simulink model "LQR01"  (Simulink 9.2)
settings: Solver=VariableStepAuto  StartTime=0.0  StopTime=60  RelTol=1e-3
libraries: Solver_SF x1, simulink x1
settings Model: Creator=GTR  LastModifiedBy=tomoyo
settings SolverCC: AlgebraicLoopSolver=LineSearch
settings DataIOCC: LimitDataPoints=off  SaveFormat=Dataset  SignalLoggingSaveFormat=Dataset
settings OptimizationCC: LifeSpan=auto
settings DebuggingCC: UnderspecifiedInitializationDetection=Simplified  MergeDetectMultiDrivingBlocksExec=error  FcnCallInpInsideContextMsg=error  StateNameClashWarn=none  SFUnexpectedBacktrackingDiag=error  SFNoUnconditionalDefaultTransitionDiag=error  SFExecutionAtInitializationDiag=warning
settings HardwareCC: ProdBitPerPointer=64  ProdBitPerSizeT=64  ProdBitPerPtrDiffT=64  ProdLargestAtomicFloat=Float  ProdIntDivRoundTo=Zero  ProdEndianess=LittleEndian  ProdWordSize=64  ProdHWDeviceType=Intel->x86-64 (Windows64)
settings ModelReferenceCC: PropagateSignalLabelsOutOfModel=on
settings SFSimCC: SimUseLocalCustomCode=on
settings RTWCC: RTWUseLocalCustomCode=on
settings CodeAppCC: StateflowObjectComments=off
settings GRTTargetCC: TargetLangStandard=C99 (ISO)  GeneratePreprocessorConditionals=Use local settings  CombineOutputUpdateFcns=on  GRTInterface=off
settings ConfigComp: CovMetricSettings=dwe  CovHtmlReporting=off  CovSaveCumulativeToWorkspaceVar=off  CovSaveSingleToWorkspaceVar=off  CovExternalEMLEnable=on

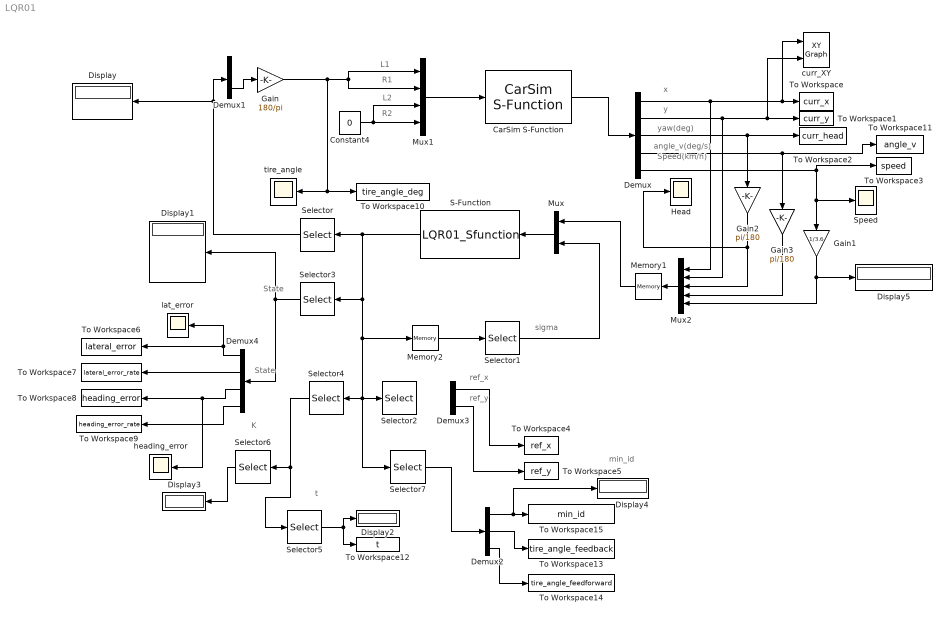
== system LQR01 ==
  note: min_id
  note: K
  note: State
  note: ref_x
  note: sigma
  note: x
  note: y
  note: yaw(deg)
  note: Speed(km/h)
  note: L1
  note: R1
  note: L2
  note: R2
  note: ref_y
  note: State
  note: angle_v(deg/s)
  note: t
  CarSim S-Function : Solver_SF/CarSim S-Function  Priority=1  VehicleCode=i_i  SIMFILE=simfile
  Constant4 : Constant  Value=0
  Demux : Demux  Outputs=5
  Demux1 : Demux  Outputs=2
  Demux2 : Demux  Outputs=3
  Demux3 : Demux  Outputs=2
  Demux4 : Demux
  Display{,1..5} (6 alike) : Display
  Gain : Gain  Gain=180/pi
  Gain1 : Gain  Gain=1/3.6
  Gain2 : Gain  Gain=pi/180
  Gain3 : Gain  Gain=pi/180
  Head : Scope
  Memory1 : Memory
  Memory2 : Memory
  Mux : Mux  Inputs=2
  Mux1 : Mux
  Mux2 : Mux  Inputs=5
  S-Function : S-Function  FunctionName=LQR01_Sfunction  SFunctionDeploymentMode=off  EnableBusSupport=off
  Selector : Selector  InputPortWidth=19  IndexOptions=Index vector (dialog)  Indices=[1 2]  OutputSizes=1
  Selector1 : Selector  InputPortWidth=19  IndexOptions=Index vector (dialog)  Indices=[2]  OutputSizes=1
  Selector2 : Selector  InputPortWidth=19  IndexOptions=Index vector (dialog)  Indices=[6 7]  OutputSizes=1
  Selector3 : Selector  InputPortWidth=19  IndexOptions=Index vector (dialog)  Indices=[8 9 10 11]  OutputSizes=1
  Selector4 : Selector  InputPortWidth=19  IndexOptions=Index vector (dialog)  Indices=[12 13 14 15 16]  OutputSizes=1
  Selector5 : Selector  InputPortWidth=5  IndexOptions=Index vector (dialog)  Indices=[5]  OutputSizes=1
  Selector6 : Selector  InputPortWidth=5  IndexOptions=Index vector (dialog)  Indices=[1 2 3 4]  OutputSizes=1
  Selector7 : Selector  InputPortWidth=19  IndexOptions=Index vector (dialog)  Indices=[17 18 19]  OutputSizes=1
  Speed : Scope
  To Workspace : ToWorkspace  VariableName=curr_x  SaveFormat=Timeseries  SampleTime=-1
  To Workspace1 : ToWorkspace  VariableName=curr_y  SaveFormat=Timeseries  SampleTime=-1
  To Workspace10 : ToWorkspace  VariableName=tire_angle_deg  SaveFormat=Timeseries  SampleTime=-1
  To Workspace11 : ToWorkspace  VariableName=angle_v  SaveFormat=Timeseries  SampleTime=-1
  To Workspace12 : ToWorkspace  VariableName=t  SaveFormat=Timeseries  SampleTime=-1
  To Workspace13 : ToWorkspace  VariableName=tire_angle_feedback  SaveFormat=Timeseries  SampleTime=-1
  To Workspace14 : ToWorkspace  VariableName=tire_angle_feedforward  SaveFormat=Timeseries  SampleTime=-1
  To Workspace15 : ToWorkspace  VariableName=min_id  SaveFormat=Timeseries  SampleTime=-1
  To Workspace2 : ToWorkspace  VariableName=curr_head  SaveFormat=Timeseries  SampleTime=-1
  To Workspace3 : ToWorkspace  VariableName=speed  SaveFormat=Timeseries  SampleTime=-1
  To Workspace4 : ToWorkspace  VariableName=ref_x  SaveFormat=Timeseries  SampleTime=-1
  To Workspace5 : ToWorkspace  VariableName=ref_y  SaveFormat=Timeseries  SampleTime=-1
  To Workspace6 : ToWorkspace  VariableName=lateral_error  SaveFormat=Timeseries  SampleTime=-1
  To Workspace7 : ToWorkspace  VariableName=lateral_error_rate  SaveFormat=Timeseries  SampleTime=-1
  To Workspace8 : ToWorkspace  VariableName=heading_error  SaveFormat=Timeseries  SampleTime=-1
  To Workspace9 : ToWorkspace  VariableName=heading_error_rate  SaveFormat=Timeseries  SampleTime=-1
  curr_XY : simulink/Sinks/XY Graph  xmin=0  xmax=150  ymin=-20  ymax=20  st=-1
  heading_error : Scope
  lat_error : Scope
  tire_angle : Scope
  wires:
  CarSim S-Function/1 -> Demux/1
  Demux/1 -> To Workspace/1, curr_XY/1, Mux2/1
  Demux/2 -> curr_XY/2, To Workspace1/1, Mux2/2
  Demux/3 -> Gain2/1, To Workspace2/1
  Constant4/1 -> Mux1/3, Mux1/4
  Mux1/1 -> CarSim S-Function/1
  S-Function/1 -> Selector/1, Memory2/1, Selector7/1, Selector4/1, Selector2/1, Selector3/1
  Demux1/2 -> Gain/1
  Selector/1 -> Demux1/1, Display/1
  Mux/1 -> S-Function/1
  Demux3/1 -> To Workspace4/1
  Demux3/2 -> To Workspace5/1
  Selector3/1 -> Demux4/1, Display1/1
  Demux4/1 -> lat_error/1, To Workspace6/1
  Demux4/2 -> To Workspace7/1
  Demux4/3 -> To Workspace8/1, heading_error/1
  Demux4/4 -> To Workspace9/1
  Selector4/1 -> Selector5/1, Selector6/1
  Memory1/1 -> Mux/1
  Mux2/1 -> Memory1/1
  Memory2/1 -> Selector1/1
  Gain2/1 -> Head/1, Mux2/3
  Demux/5 -> To Workspace3/1, Gain1/1, Speed/1
  Demux/4 -> Gain3/1, To Workspace11/1
  Gain3/1 -> Mux2/4
  Gain1/1 -> Display5/1, Mux2/5
  Selector1/1 -> Mux/2
  Gain/1 -> To Workspace10/1, tire_angle/1, Mux1/1, Mux1/2
  Selector6/1 -> Display3/1
  Selector5/1 -> Display2/1, To Workspace12/1
  Selector7/1 -> Demux2/1
  Demux2/1 -> Display4/1, To Workspace15/1
  Demux2/2 -> To Workspace13/1
  Demux2/3 -> To Workspace14/1
